simulink library "cubex_simulation"  (R2016a)
settings: Solver=ode45  StartTime=0.0  StopTime=10.0  RelTol=1e-3
undefined symbols (not defined in the file or in its folder): motor, wheel
libraries: simulink x1
settings Model: Creator=Love  LastModifiedBy=Love
settings DataIOCC: LimitDataPoints=on
settings DebuggingCC: AllowSymbolicDim=off

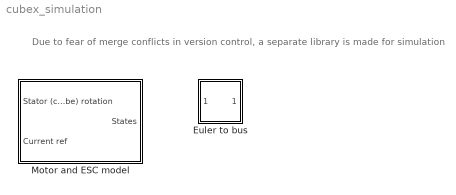
== system cubex_simulation ==
  note: Due to fear of merge conflicts in version control, a separate library is made for simulation
  Euler to bus : Subsystem
  Motor and ESC model : Subsystem

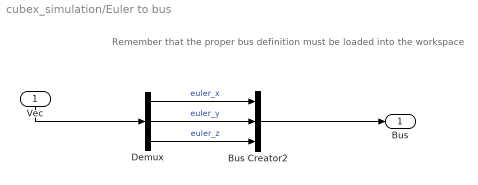
== system cubex_simulation/Euler to bus ==
  note: Remember that the proper bus definition must be loaded into the workspace
  Vec : Inport
  Bus Creator2 : BusCreator  Inputs='euler_x','euler_y','euler_z'  OutDataTypeStr=Bus: euler
  Demux : Demux  Outputs=3
  Bus : Outport
  wires:
  Bus Creator2/1 -> Bus/1
  Demux/1 -> Bus Creator2/1  "euler_x"
  Vec/1 -> Demux/1
  Demux/3 -> Bus Creator2/3  "euler_z"
  Demux/2 -> Bus Creator2/2  "euler_y"

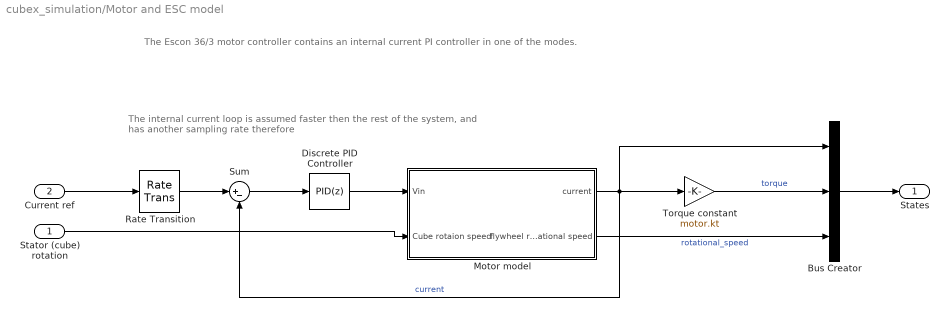
== system cubex_simulation/Motor and ESC model ==
  note: The Escon 36/3 motor controller contains an internal current PI controller in one of the modes.
  note: The internal current loop is assumed faster then the rest of the system, and has another sampling rate therefore
  Stator (cube) rotation : Inport
  Current ref : Inport  Port=2
  Bus Creator : BusCreator  Inputs='current','torque','rotational_speed'  OutDataTypeStr=Bus: motorStates
  Discrete PID Controller : simulink/Continuous/PID Controller  Controller=PID  TimeDomain=Discrete-time  SampleTime=0.001  IntegratorMethod=Forward Euler  FilterMethod=Forward Euler  Form=Parallel  UseFilter=on  ControllerParametersSource=internal  P=4.86484791836619  I=892.83595159061  D=-3.51372671337991e-05  N=1968.68827759537  InitialConditionSource=internal  InitialConditionForIntegrator=0  InitialConditionForFilter=0  ExternalReset=none  LimitOutput=on  UpperSaturationLimit=motor.Vbat  LowerSaturationLimit=-motor.Vbat  LinearizeAsGain=on  AntiWindupMode=clamping  Kb=1  TrackingMode=off  Kt=1  PParamMin=[]  PParamMax=[]  IParamMin=[]  IParamMax=[]  DParamMin=[]  DParamMax=[]  NParamMin=[]  NParamMax=[]  KbParamMin=[]  KbParamMax=[]  KtParamMin=[]  KtParamMax=[]  POutMin=[]  POutMax=[]  IOutMin=[]  IOutMax=[]  DOutMin=[]  DOutMax=[]  NOutMin=[]  NOutMax=[]  KbOutMin=[]  KbOutMax=[]  KtOutMin=[]  KtOutMax=[]  IntegratorOutMin=[]  IntegratorOutMax=[]  FilterOutMin=[]  FilterOutMax=[]  SumOutMin=[]  SumOutMax=[]  SumI1OutMin=[]  SumI1OutMax=[]  SumI2OutMin=[]  SumI2OutMax=[]  SumI3OutMin=[]  SumI3OutMax=[]  SumDOutMin=[]  SumDOutMax=[]  SaturationOutMin=[]  SaturationOutMax=[]  IntegratorContinuousStateAttributes=''  IntegratorStateMustResolveToSignalObject=off  IntegratorRTWStateStorageClass=Auto  FilterContinuousStateAttributes=''  FilterStateMustResolveToSignalObject=off  FilterRTWStateStorageClass=Auto  DifferentiatorICPrevScaledInput=0  DifferentiatorOutMin=[]  DifferentiatorOutMax=[]
  Motor model : Subsystem
  Rate Transition : RateTransition  OutPortSampleTime=0.001
  Sum : Sum  Inputs=|+-
  Torque constant : Gain  Gain=motor.kt
  "States " : Outport  OutDataTypeStr=Bus: motorStates
  wires:
  Motor model/1(current) -> Bus Creator/1, Sum/2, Torque constant/1  "current"
  Torque constant/1 -> Bus Creator/2  "torque"
  Sum/1 -> Discrete PID Controller/1
  Rate Transition/1 -> Sum/1
  Discrete PID Controller/1 -> Motor model/1(Vin)
  Current ref/1 -> Rate Transition/1
  Stator (cube) rotation/1 -> Motor model/2(Cube rotaion speed)
  Motor model/2(flywheel rotational speed) -> Bus Creator/3  "rotational_speed"
  Bus Creator/1 -> "States "/1

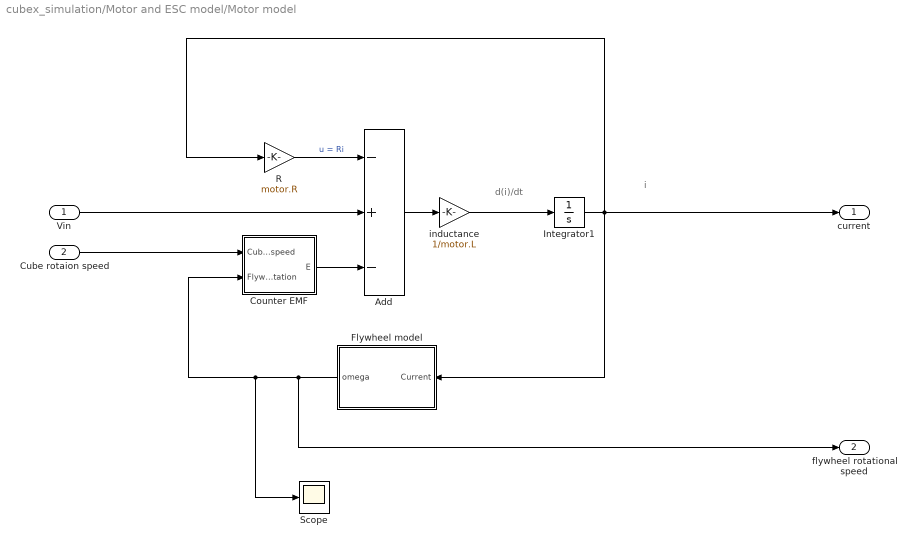
== system cubex_simulation/Motor and ESC model/Motor model ==
  note: i
  note: d(i)/dt
  Vin : Inport
  Cube rotaion speed : Inport  Port=2
  Add : Sum  Inputs=-+-
  Counter EMF : Subsystem
  Flywheel model : Subsystem
  Integrator1 : Integrator
  R : Gain  Gain=motor.R
  Scope : Scope
  inductance : Gain  Gain=1/motor.L
  current : Outport
  flywheel rotational speed : Outport  Port=2
  wires:
  inductance/1 -> Integrator1/1
  Add/1 -> inductance/1
  R/1 -> Add/1  "u = Ri"
  Integrator1/1 -> current/1, Flywheel model/1(Current), R/1
  Vin/1 -> Add/2
  Cube rotaion speed/1 -> Counter EMF/1(Cube rot speed)
  Flywheel model/1(omega) -> flywheel rotational speed/1, Scope/1, Counter EMF/2(Flywheel rotation)
  Counter EMF/1(E) -> Add/3

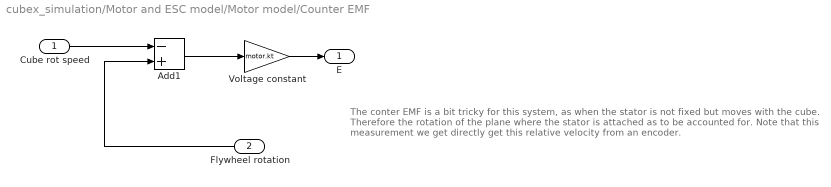
== system cubex_simulation/Motor and ESC model/Motor model/Counter EMF ==
  note: The conter EMF is a bit tricky for this system, as when the stator is not fixed but moves with the cube. Therefore the rotation of the plane
      | where the stator is attached as to  be accounted for.
      |
      | Note that this measurement we get directly get this relative velocity from an encoder.
  Cube rot speed : Inport
  Flywheel rotation : Inport  Port=2
  Add1 : Sum  Inputs=-+
  Voltage constant : Gain  Gain=motor.kt
  E : Outport
  wires:
  Cube rot speed/1 -> Add1/1
  Flywheel rotation/1 -> Add1/2
  Add1/1 -> Voltage constant/1
  Voltage constant/1 -> E/1

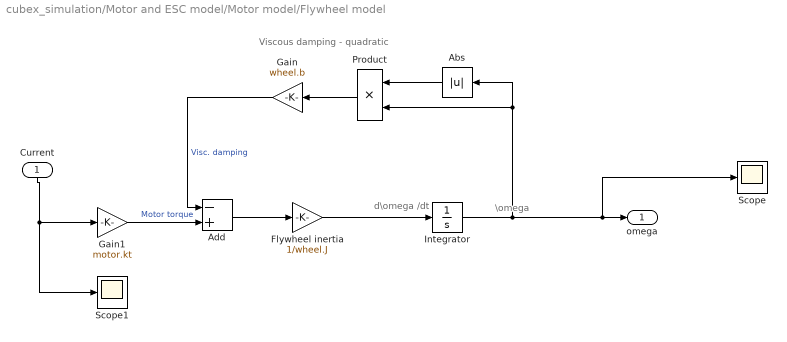
== system cubex_simulation/Motor and ESC model/Motor model/Flywheel model ==
  note: Viscous damping - quadratic
  note: \omega
  note: d\omega /dt
  Current : Inport
  Abs : Abs
  Add : Sum  Inputs=-+
  Flywheel inertia : Gain  Gain=1/wheel.J
  Gain : Gain  Gain=wheel.b
  Gain1 : Gain  Gain=motor.kt
  Integrator : Integrator
  Product : Product
  Scope : Scope
  Scope1 : Scope
  omega : Outport
  wires:
  Current/1 -> Gain1/1, Scope1/1
  Flywheel inertia/1 -> Integrator/1
  Add/1 -> Flywheel inertia/1
  Gain1/1 -> Add/2  "Motor torque"
  Gain/1 -> Add/1  "Visc. damping"
  Abs/1 -> Product/1
  Integrator/1 -> Scope/1, omega/1, Abs/1, Product/2
  Product/1 -> Gain/1
